simulink model "Simulink_Simulation"  (Simulink 10.1)
settings: Solver=ode23t  StartTime=0.0  StopTime=0.6  RelTol=1e-3  EnableMultiTasking=on
libraries: powerlib x15, powerlib_meascontrol x2
settings Model: Creator=asus1  LastModifiedBy=x64
settings DataIOCC: LimitDataPoints=on
settings DebuggingCC: UnderspecifiedInitializationDetection=Simplified  MergeDetectMultiDrivingBlocksExec=error  SolverPrmCheckMsg=warning
settings GRTTargetCC: CombineOutputUpdateFcns=on  GRTInterface=off
settings ConfigComp: CovSFcnEnable=off
settings SimscapeCC: SimscapeNormalizeSystem=off

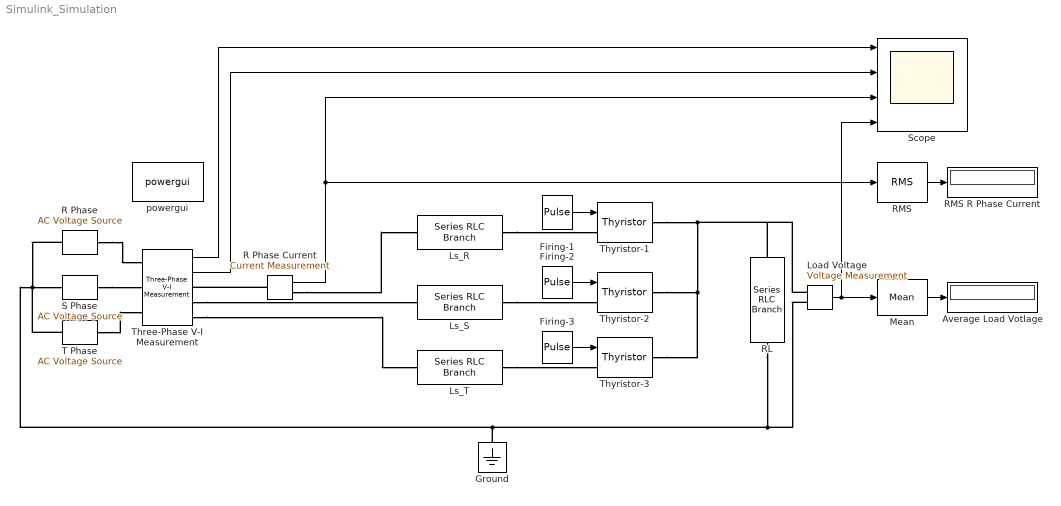
== system Simulink_Simulation ==
  " RMS R Phase Current" : Display
      settings: Format=bank
  Average Load Votlage : Display
  Firing-1 : DiscretePulseGenerator  PulseType=Time based  Amplitude=5  Period=0.02  PulseWidth=50  PhaseDelay=0.02/6
  Firing-2 : DiscretePulseGenerator  PulseType=Time based  Amplitude=5  Period=0.02  PulseWidth=50  PhaseDelay=0.01
  Firing-3 : DiscretePulseGenerator  PulseType=Time based  Amplitude=5  Period=0.02  PulseWidth=50  PhaseDelay=6/360
  Ground : powerlib/Elements/Ground  LConnTagsString=a
  Load Voltage : powerlib/Measurements/Voltage Measurement  PhasorSimulation=off  OutputType=Complex  PSBequivalent=0
  Ls_R : powerlib/Elements/Series RLC Branch  LConnTagsString=__new0  RConnTagsString=__new0  BranchType=L  Resistance=1  Inductance=1e-2  SetiL0=off  InitialCurrent=0  Capacitance=1e-6  Setx0=off  InitialVoltage=0  Measurements=None
  Ls_S : powerlib/Elements/Series RLC Branch  LConnTagsString=__new0  RConnTagsString=__new0  BranchType=L  Resistance=1  Inductance=1e-2  SetiL0=off  InitialCurrent=0  Capacitance=1e-6  Setx0=off  InitialVoltage=0  Measurements=None
  Ls_T : powerlib/Elements/Series RLC Branch  LConnTagsString=__new0  RConnTagsString=__new0  BranchType=L  Resistance=1  Inductance=1e-2  SetiL0=off  InitialCurrent=0  Capacitance=1e-6  Setx0=off  InitialVoltage=0  Measurements=None
  Mean : powerlib_meascontrol/Measurements/Mean  Freq=50  Vinit=0  Ts=0
  R Phase : powerlib/Electrical Sources/AC Voltage Source  Amplitude=(380/sqrt(3))*sqrt(2)  Phase=0  Frequency=50  SampleTime=0  Measurements=None  BusType=swing  Pref=10e3  Qref=0  Qmin=-inf  Qmax=+inf
  R Phase Current : powerlib/Measurements/Current Measurement  PhasorSimulation=off  OutputType=Complex  PSBequivalent=0
  RL : powerlib/Elements/Series RLC Branch  LConnTagsString=__new0  RConnTagsString=__new0  BranchType=RL  Resistance=9.645  Inductance=1  SetiL0=off  InitialCurrent=0  Capacitance=1e-6  Setx0=off  InitialVoltage=0  Measurements=None
  RMS : powerlib_meascontrol/Measurements/RMS  TrueRMS=on  Freq=50  RMSInit=0  Ts=0
  S Phase : powerlib/Electrical Sources/AC Voltage Source  Amplitude=(380/sqrt(3))*sqrt(2)  Phase=-120  Frequency=50  SampleTime=0  Measurements=None  BusType=swing  Pref=10e3  Qref=0  Qmin=-inf  Qmax=+inf
  "Scope " : Scope  NumInputPorts=4
  T Phase : powerlib/Electrical Sources/AC Voltage Source  Amplitude=(380/sqrt(3))*sqrt(2)  Phase=120  Frequency=50  SampleTime=0  Measurements=None  BusType=swing  Pref=10e3  Qref=0  Qmin=-inf  Qmax=+inf
  "Three-Phase V-I Measurement " : powerlib/Measurements/Three-Phase V-I Measurement  VoltageMeasurement=phase-to-ground  SetLabelV=off  LabelV=Vabc  Vpu=off  VpuLL=off  CurrentMeasurement=yes  SetLabelI=off  LabelI=Iabc  Ipu=off  Pbase=100e6  Vbase=500e3  OutputType=Complex  PhasorSimulation=off  PSBequivalent=0
  Thyristor-1 : powerlib/Power Electronics/Thyristor  Ron=0.000001  Lon=0  Vf=0  IC=0  Rs=5000  Cs=250e-3  Measurements=off
  Thyristor-2 : powerlib/Power Electronics/Thyristor  Ron=0.000001  Lon=0  Vf=0  IC=0  Rs=5000  Cs=250e-3  Measurements=off
  Thyristor-3 : powerlib/Power Electronics/Thyristor  Ron=0.000001  Lon=0  Vf=0  IC=0  Rs=5000  Cs=250e-3  Measurements=off
  powergui : powerlib/powergui  Priority=1  SimulationMode=Discrete  SampleTime=5e-006  frequency=60  Iterations=50  frequencyindice=50  Pbase=1000e6  ErrMax=1e-4  UnitsV=kV  UnitsW=MW  buscounter=0  FunctionMessages=off  echomessages=off  EnableUseOfTLC=off  CurrentSourceSwitches=off  DisableSnubberDevices=off  DisableRonSwitches=off  DisableVfSwitches=off  DisplayEquations=off  AutomaticDiscreteSolvers=off  SolverType=Tustin  Interpol=off  ExternalGateDelay=off  methode=off  Ts=100  x0status=blocks  SPID=off  SwTol=0  HookPort=off  NonlinearTolerance=1e-4  nMaxIteration=100  ContinueOnMaxIteration=off  RestoreLinks=warning  ResistiveCurrentMeasurement=off  Frange=[0:2:500]  Ylog=off  Xlog=on  ShowGrid=off  save=off  variable=ZData  structure=0  ZoomFFT=off  StartTime=0.0  cycles=1  DisplayStyle=1  fundamental=60  FreqAxis=off  MaxFrequency=1000  frequencyindicesteady=1  RmsSteady=1  display=off
  wires:
  R Phase Current/1 -> RMS/1, "Scope "/3
  RMS/1 -> " RMS R Phase Current"/1
  Firing-1/1 -> Thyristor-1/1
  Firing-2/1 -> Thyristor-2/1
  Firing-3/1 -> Thyristor-3/1
  Load Voltage/1 -> "Scope "/4, Mean/1
  Mean/1 -> Average Load Votlage/1
  "Three-Phase V-I Measurement "/2 -> "Scope "/2
  "Three-Phase V-I Measurement "/1 -> "Scope "/1
  connections:
  Thyristor-2/RConn1 -- Thyristor-3/RConn1 -- Thyristor-1/RConn1 -- Load Voltage/LConn1 -- RL/LConn1
  Ls_T/RConn1 -- Thyristor-3/LConn1
  Ls_R/RConn1 -- Thyristor-1/LConn1
  Ls_S/RConn1 -- Thyristor-2/LConn1
  "Three-Phase V-I Measurement "/RConn2 -- Ls_S/LConn1
  R Phase Current/RConn1 -- Ls_R/LConn1
  R Phase/RConn1 -- "Three-Phase V-I Measurement "/LConn1
  S Phase/RConn1 -- "Three-Phase V-I Measurement "/LConn2
  T Phase/RConn1 -- "Three-Phase V-I Measurement "/LConn3
  R Phase Current/LConn1 -- "Three-Phase V-I Measurement "/RConn1
  "Three-Phase V-I Measurement "/RConn3 -- Ls_T/LConn1
  Load Voltage/LConn2 -- RL/RConn1 -- T Phase/LConn1 -- S Phase/LConn1 -- R Phase/LConn1 -- Ground/LConn1
